simulink model "control_system"  (R2017b)
settings: Solver=VariableStepAuto  StartTime=0.0  StopTime=3  RelTol=1e-3
values from neighbouring files (symbols this model uses):
  alpha = 1/(I_sp*g)    (= 0.00045305244082)    [parameters.m]
  g = 9.81    [parameters.m]
  I_sp = 225    [parameters.m]
  m_0 = 1905    [parameters.m]
libraries: simulink x1
settings Model: Creator=malyuta  LastModifiedBy=malyuta

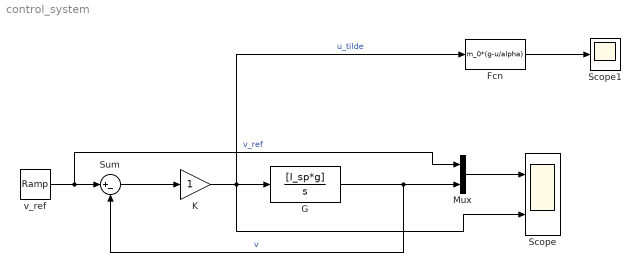
== system control_system ==
  Fcn : Fcn  Expr=m_0*(g-u/alpha)
  G : TransferFcn  Numerator=[I_sp*g]  Denominator=[1 0]
  K : Gain
  Mux : Mux  Inputs=2
  Scope : Scope  NumInputPorts=2
  Scope1 : Scope
  Sum : Sum  Inputs=|+-
  v_ref : simulink/Sources/Ramp  slope=-70  start=2  X0=0
  wires:
  K/1 -> Fcn/1, Scope/2, G/1  "u_tilde"
  Sum/1 -> K/1
  G/1 -> Mux/2, Sum/2  "v"
  v_ref/1 -> Mux/1, Sum/1  "v_ref"
  Mux/1 -> Scope/1
  Fcn/1 -> Scope1/1
